simulink model "FOC_SMPMSM_SPWM"  (R2019a)
settings: Solver=VariableStepAuto  StartTime=0.0  StopTime=1  RelTol=1e-3
values from neighbouring files (symbols this model uses):
  Lq = 0.000165    [FOC_Parameters.mat]
  PM_flux = 0.11    [FOC_Parameters.mat]
  pp = 4    [FOC_Parameters.mat]
  Rs = 0.016    [FOC_Parameters.mat]
libraries: simulink x4, powerlib x3, electricdrivelib x1, powerlib_meascontrol x1
settings Model: Creator=ryusl  LastModifiedBy=ryusl

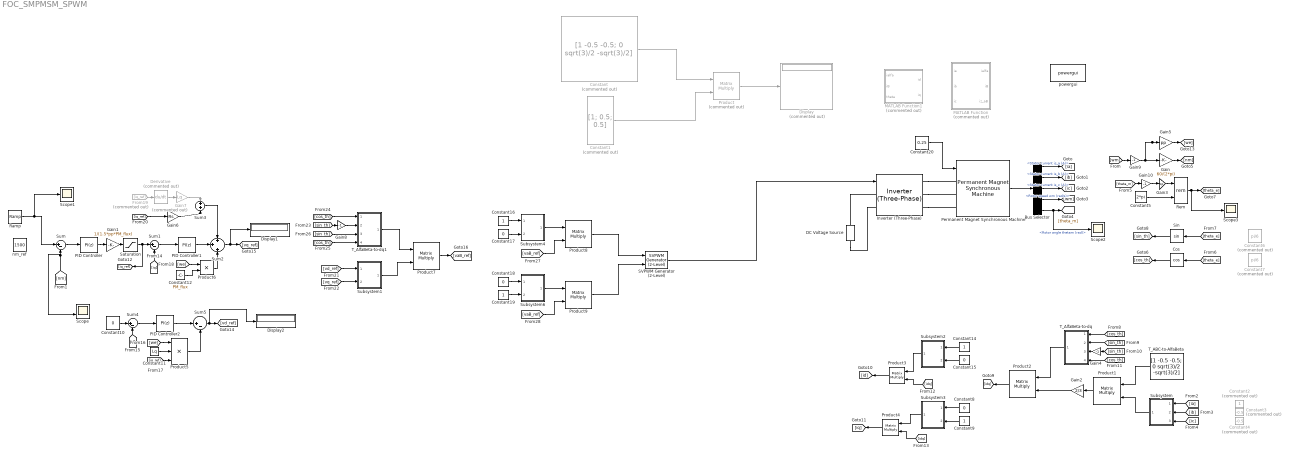
== system FOC_SMPMSM_SPWM ==
  Bus Selector : BusSelector  OutputSignals=Stator current is_a (A),Stator current is_b (A),Stator current is_c (A),Rotor speed wm (rad/s),Rotor angle thetam (rad)
  Constant : Constant  Commented=on  Value=[1 -0.5 -0.5; 0 sqrt(3)/2 -sqrt(3)/2]  VectorParams1D=off
  Constant1 : Constant  Commented=on  Value=[1; 0.5; 0.5]  VectorParams1D=off
  Constant{8,10,15,17..18} (5 alike) : Constant  Value=0
  Constant11 : Constant  Value=Lq
  Constant12 : Constant  Value=PM_flux
  Constant{9,14,16,19} (4 alike) : Constant
  Constant2 : Constant  Commented=on
  Constant20 : Constant  Value=0.25
  Constant3 : Constant  Commented=on  Value=-0.5
  Constant4 : Constant  Commented=on  Value=-0.5
  Constant5 : Constant  Value=2*pi
  Constant6 : Constant  Commented=on  Value=pi/6
  Constant7 : Constant  Commented=on  Value=pi/6
  Cos : Trigonometry  Operator=cos
  DC Voltage Source : powerlib/Electrical Sources/DC Voltage Source  Amplitude=600  Measurements=None
      settings: SourceProductName=Simscape Electrical
  Derivative : Derivative  Commented=on
  Display : Display  Commented=on
  Display1 : Display
  Display2 : Display
  From19 : From  Commented=on  GotoTag=iq_ref
  Gain : Gain  Gain=60/(2*pi)
  Gain1 : Gain  Gain=1/(1.5*pp*PM_flux)
  Gain{4,8..10} (4 alike) : Gain  Gain=-1
  Gain2 : Gain  Gain=2/3
  Gain3 : Gain  Gain=pp
  Gain5 : Gain  Gain=pp
  Gain6 : Gain  Gain=Rs
  Gain7 : Gain  Commented=on  Gain=Lq
  Inverter (Three-Phase) : electricdrivelib/Fundamental Drive Blocks/Inverter (Three-Phase)  LabelModeActiveChoice=Detailed  detailLevel=Detailed  driveType=Field-oriented control  Ts=2e-6  SnubberResistance=10e3  SnubberCapacitance=inf  Device=IGBT / Diodes  Ron=1e-3  ForwardVoltages=[1.2,1.2]  GTOparameters=[1e-6,2e-6]  IGBTparameters=[1e-6,2e-6]  Measurements=All voltages and currents  converterType=Inverter  SourceFrequency=60  ReferenceFrame=Rotor  dqInductances=[8.5e-3,8.5e-3]  Inductance=8.5e-3  Ls=0  Resistance=0.2  Flux=0.175  Stator_sm=[2.01e-3,4.289e-4,4.477e-3,1.354e-3]  Stator_im=[14.85e-3,0.3027e-3]  Rotor=[9.295e-3,0.3027e-3]  Lm=10.46e-3  p=4
      settings: AttributesFormatString=%<BlockChoice>  SourceProductName=Simscape Electrical  SourceProductBaseCode=PS
  MATLAB Function : MATLAB Function  Commented=on  TreatAsAtomicUnit=on
  MATLAB Function1 : MATLAB Function  Commented=on  TreatAsAtomicUnit=on
  PID Controller : simulink/Continuous/PID Controller  Controller=PI  Form=Parallel  TimeDomain=Discrete-time  SampleTime=-1  IntegratorMethod=Forward Euler  FilterMethod=Forward Euler  ControllerParametersSource=internal  P=10  I=2  D=0  UseFilter=on  N=100  TunerSelectOption=Transfer Function Based (PID Tuner App)  InitialConditionSource=internal  InitialConditionForIntegrator=0  InitialConditionForFilter=0  DifferentiatorICPrevScaledInput=0  ExternalReset=none  TrackingMode=off  Kt=1  LimitOutput=off  UpperSaturationLimit=inf  LowerSaturationLimit=-inf  LinearizeAsGain=on  AntiWindupMode=none  Kb=1  POutMin=[]  POutMax=[]  IOutMin=[]  IOutMax=[]  DOutMin=[]  DOutMax=[]  NOutMin=[]  NOutMax=[]  SumOutMin=[]  SumOutMax=[]  SaturationOutMin=[]  SaturationOutMax=[]  PParamMin=[]  PParamMax=[]  IParamMin=[]  IParamMax=[]  DParamMin=[]  DParamMax=[]  NParamMin=[]  NParamMax=[]  KbParamMin=[]  KbParamMax=[]  KtParamMin=[]  KtParamMax=[]  KbOutMin=[]  KbOutMax=[]  KtOutMin=[]  KtOutMax=[]  IntegratorOutMin=[]  IntegratorOutMax=[]  FilterOutMin=[]  FilterOutMax=[]  SumI1OutMin=[]  SumI1OutMax=[]  SumI2OutMin=[]  SumI2OutMax=[]  SumI3OutMin=[]  SumI3OutMax=[]  SumI4OutMin=[]  SumI4OutMax=[]  SumDOutMin=[]  SumDOutMax=[]  DifferentiatorOutMin=[]  DifferentiatorOutMax=[]  FilterDiffOutCoefMin=[]  FilterDiffOutCoefMax=[]  ReciprocalOutMin=[]  ReciprocalOutMax=[]  SumDenOutMin=[]  SumDenOutMax=[]  SumNumOutMin=[]  SumNumOutMax=[]  DivideOutMin=[]  DivideOutMax=[]  IntegratorContinuousStateAttributes=''  IntegratorStateMustResolveToSignalObject=off  IntegratorRTWStateStorageClass=Auto  FilterContinuousStateAttributes=''  FilterStateMustResolveToSignalObject=off  FilterRTWStateStorageClass=Auto  ParallelPVariant=InternalParameters  IdealPVariant=Disabled  IVariant=InternalParameters  DVariant=Disabled  IntegratorVariant=Discrete  SatVariant=Disabled  AWVariant=Passthrough  PCopyVariant=Disabled  TRVariant=Disabled  FdbkBlocksVariant=Forward  IdealPFdbkVariant=Disabled  SatFdbkVariant=Disabled  DerivativeFilterVariant=Disabled  NVariant=Disabled  NCopyVariant=Disabled_SignalSpec  FilterICVariant=Disabled  IntegratorICVariant=InternalICs  ExternalResetVariant=Disabled  TRSumVariant=Passthrough  SumFdbkVariant=Disabled  SumVariant=Sum_PI
  PID Controller1 : simulink/Continuous/PID Controller  Controller=PI  Form=Parallel  TimeDomain=Discrete-time  SampleTime=-1  IntegratorMethod=Forward Euler  FilterMethod=Forward Euler  ControllerParametersSource=internal  P=5  I=0.5  D=0  UseFilter=on  N=100  TunerSelectOption=Transfer Function Based (PID Tuner App)  InitialConditionSource=internal  InitialConditionForIntegrator=0  InitialConditionForFilter=0  DifferentiatorICPrevScaledInput=0  ExternalReset=none  TrackingMode=off  Kt=1  LimitOutput=off  UpperSaturationLimit=inf  LowerSaturationLimit=-inf  LinearizeAsGain=on  AntiWindupMode=none  Kb=1  POutMin=[]  POutMax=[]  IOutMin=[]  IOutMax=[]  DOutMin=[]  DOutMax=[]  NOutMin=[]  NOutMax=[]  SumOutMin=[]  SumOutMax=[]  SaturationOutMin=[]  SaturationOutMax=[]  PParamMin=[]  PParamMax=[]  IParamMin=[]  IParamMax=[]  DParamMin=[]  DParamMax=[]  NParamMin=[]  NParamMax=[]  KbParamMin=[]  KbParamMax=[]  KtParamMin=[]  KtParamMax=[]  KbOutMin=[]  KbOutMax=[]  KtOutMin=[]  KtOutMax=[]  IntegratorOutMin=[]  IntegratorOutMax=[]  FilterOutMin=[]  FilterOutMax=[]  SumI1OutMin=[]  SumI1OutMax=[]  SumI2OutMin=[]  SumI2OutMax=[]  SumI3OutMin=[]  SumI3OutMax=[]  SumI4OutMin=[]  SumI4OutMax=[]  SumDOutMin=[]  SumDOutMax=[]  DifferentiatorOutMin=[]  DifferentiatorOutMax=[]  FilterDiffOutCoefMin=[]  FilterDiffOutCoefMax=[]  ReciprocalOutMin=[]  ReciprocalOutMax=[]  SumDenOutMin=[]  SumDenOutMax=[]  SumNumOutMin=[]  SumNumOutMax=[]  DivideOutMin=[]  DivideOutMax=[]  IntegratorContinuousStateAttributes=''  IntegratorStateMustResolveToSignalObject=off  IntegratorRTWStateStorageClass=Auto  FilterContinuousStateAttributes=''  FilterStateMustResolveToSignalObject=off  FilterRTWStateStorageClass=Auto  ParallelPVariant=InternalParameters  IdealPVariant=Disabled  IVariant=InternalParameters  DVariant=Disabled  IntegratorVariant=Discrete  SatVariant=Disabled  AWVariant=Passthrough  PCopyVariant=Disabled  TRVariant=Disabled  FdbkBlocksVariant=Forward  IdealPFdbkVariant=Disabled  SatFdbkVariant=Disabled  DerivativeFilterVariant=Disabled  NVariant=Disabled  NCopyVariant=Disabled_SignalSpec  FilterICVariant=Disabled  IntegratorICVariant=InternalICs  ExternalResetVariant=Disabled  TRSumVariant=Passthrough  SumFdbkVariant=Disabled  SumVariant=Sum_PI
  PID Controller2 : simulink/Continuous/PID Controller  Controller=PI  Form=Parallel  TimeDomain=Discrete-time  SampleTime=-1  IntegratorMethod=Forward Euler  FilterMethod=Forward Euler  ControllerParametersSource=internal  P=5  I=0.5  D=0  UseFilter=on  N=100  TunerSelectOption=Transfer Function Based (PID Tuner App)  InitialConditionSource=internal  InitialConditionForIntegrator=0  InitialConditionForFilter=0  DifferentiatorICPrevScaledInput=0  ExternalReset=none  TrackingMode=off  Kt=1  LimitOutput=off  UpperSaturationLimit=inf  LowerSaturationLimit=-inf  LinearizeAsGain=on  AntiWindupMode=none  Kb=1  POutMin=[]  POutMax=[]  IOutMin=[]  IOutMax=[]  DOutMin=[]  DOutMax=[]  NOutMin=[]  NOutMax=[]  SumOutMin=[]  SumOutMax=[]  SaturationOutMin=[]  SaturationOutMax=[]  PParamMin=[]  PParamMax=[]  IParamMin=[]  IParamMax=[]  DParamMin=[]  DParamMax=[]  NParamMin=[]  NParamMax=[]  KbParamMin=[]  KbParamMax=[]  KtParamMin=[]  KtParamMax=[]  KbOutMin=[]  KbOutMax=[]  KtOutMin=[]  KtOutMax=[]  IntegratorOutMin=[]  IntegratorOutMax=[]  FilterOutMin=[]  FilterOutMax=[]  SumI1OutMin=[]  SumI1OutMax=[]  SumI2OutMin=[]  SumI2OutMax=[]  SumI3OutMin=[]  SumI3OutMax=[]  SumI4OutMin=[]  SumI4OutMax=[]  SumDOutMin=[]  SumDOutMax=[]  DifferentiatorOutMin=[]  DifferentiatorOutMax=[]  FilterDiffOutCoefMin=[]  FilterDiffOutCoefMax=[]  ReciprocalOutMin=[]  ReciprocalOutMax=[]  SumDenOutMin=[]  SumDenOutMax=[]  SumNumOutMin=[]  SumNumOutMax=[]  DivideOutMin=[]  DivideOutMax=[]  IntegratorContinuousStateAttributes=''  IntegratorStateMustResolveToSignalObject=off  IntegratorRTWStateStorageClass=Auto  FilterContinuousStateAttributes=''  FilterStateMustResolveToSignalObject=off  FilterRTWStateStorageClass=Auto  ParallelPVariant=InternalParameters  IdealPVariant=Disabled  IVariant=InternalParameters  DVariant=Disabled  IntegratorVariant=Discrete  SatVariant=Disabled  AWVariant=Passthrough  PCopyVariant=Disabled  TRVariant=Disabled  FdbkBlocksVariant=Forward  IdealPFdbkVariant=Disabled  SatFdbkVariant=Disabled  DerivativeFilterVariant=Disabled  NVariant=Disabled  NCopyVariant=Disabled_SignalSpec  FilterICVariant=Disabled  IntegratorICVariant=InternalICs  ExternalResetVariant=Disabled  TRSumVariant=Passthrough  SumFdbkVariant=Disabled  SumVariant=Sum_PI
  Permanent Magnet Synchronous Machine : powerlib/Machines/Permanent Magnet Synchronous Machine  NbPhases=3  FluxDistribution=Sinusoidal  RotorType=Round  MechanicalLoad=Torque Tm  PresetModel=No  ShowDetailedParameters=on  MeasurementBus=off  Resistance=Rs  Inductance=8.5e-3  dqInductances=[8.5e-3,8.5e-3]  La=Ld  MachineConstant=Flux linkage established by magnets (V.s)  Flux=PM_flux  VoltageCst=79.8072  TorqueCst=0.66  Flat=120  Mechanical=[0.0027 0.0004924 pp 0]  PolePairs=4  InitialConditions=[0,0, 0,0]  InitialConditions5ph=[0 0 0 0 0 0]  TsPowergui=0  TsBlock=-1  RefAngle=90 degrees behind phase A axis (modified Park)
  Product : Product  Commented=on  Multiplication=Matrix(*)
  Product{1..4,7..9} (7 alike) : Product  Multiplication=Matrix(*)
  Product5 : Product  Inputs=3
  Product6 : Product
  Ramp : simulink/Sources/Ramp  slope=1000  start=0  InitialOutput=0
  Rem : Math  Operator=rem  SaturateOnIntegerOverflow=on
  SVPWM Generator (2-Level) : powerlib_meascontrol/Pulse & Signal Generators/SVPWM Generator (2-Level)  InputType=alpha-beta components  SwitchingPattern=Pattern #1  Fc=2000  ParUref=[0.8 -30 50]  Ts=0
      settings: SourceProductName=Simscape Electrical  SourceProductBaseCode=PS
  Saturation : Saturate  UpperLimit=500  LowerLimit=0
  Scope : Scope  NumInputPorts=2
  Scope1 : Scope
  Scope2 : Scope
  Scope3 : Scope
  Sin : Trigonometry
  Subsystem : Subsystem
  Subsystem1 : Subsystem
  Subsystem2 : Subsystem
  Subsystem3 : Subsystem
  Subsystem4 : Subsystem
  Subsystem6 : Subsystem
  Sum{,1,4..5} (4 alike) : Sum  Inputs=|+-
  Sum2 : Sum  Inputs=+|+|+
  Sum3 : Sum  Inputs=+|+
  T_ABC-to-AlfaBeta : Constant  Value=[1 -0.5 -0.5; 0 sqrt(3)/2 -sqrt(3)/2]  VectorParams1D=off
  T_AlfaBeta-to-dq : Subsystem
  T_AlfaBeta-to-dq1 : Subsystem
  nm_ref : Constant  Value=1500
  powergui : powerlib/powergui  Priority=1  SimulationMode=Discrete  SampleTime=1e-6  frequency=60  Iterations=50  frequencyindice=0  Pbase=100e6  ErrMax=1e-4  UnitsV=kV  UnitsW=MW  buscounter=0  FunctionMessages=off  echomessages=off  EnableUseOfTLC=off  CurrentSourceSwitches=off  DisableSnubberDevices=off  DisableRonSwitches=off  DisableVfSwitches=off  DisplayEquations=off  AutomaticDiscreteSolvers=off  SolverType=Tustin/Backward Euler (TBE)  Interpol=off  ExternalGateDelay=off  methode=off  Ts=100  x0status=blocks  SPID=on  SwTol=0  HookPort=off  NonlinearTolerance=0  nMaxIteration=15  ContinueOnMaxIteration=off  RestoreLinks=warning  ResistiveCurrentMeasurement=off  Frange=[0:2:500]  Ylog=off  Xlog=on  ShowGrid=off  save=off  variable=ZData  structure=0  ZoomFFT=off  StartTime=0.0  cycles=1  DisplayStyle=1  fundamental=60  FreqAxis=off  MaxFrequency=1000  frequencyindicesteady=1  RmsSteady=1  display=off
      settings: SourceProductName=Simscape Electrical
  wires:
  Constant/1 -> Product/1
  Constant1/1 -> Product/2
  Product/1 -> Display/1
  Permanent Magnet Synchronous Machine/1 -> Bus Selector/1
  Bus Selector/1 -> [ia]  "<Stator current is_a (A)>"
  Bus Selector/2 -> [ib]  "<Stator current is_b (A)>"
  Bus Selector/3 -> [ic]  "<Stator current is_c (A)>"
  Bus Selector/4 -> [wm]  "<Rotor speed wm (rad/s)>"
  Bus Selector/5 -> Scope2/1, [theta_m]  "<Rotor angle thetam (rad)>"
  Gain/1 -> [nm]
  Sum/1 -> PID Controller/1
  [nm] -> Scope/2, Sum/2
  PID Controller/1 -> Gain1/1
  T_ABC-to-AlfaBeta/1 -> Product1/1
  Subsystem/1(Matrix) -> Product1/2
  Product1/1 -> Gain2/1
  Constant5/1 -> Rem/2
  Gain3/1 -> Rem/1
  Rem/1 -> Scope3/1, [theta_e]
  Cos/1 -> [cos_th]
  Sin/1 -> [sin_th]
  Gain4/1 -> T_AlfaBeta-to-dq/3(M21)
  [cos_th] -> T_AlfaBeta-to-dq/1(M11)
  [sin_th] -> T_AlfaBeta-to-dq/2(M12)
  [sin_th] -> Gain4/1
  [cos_th] -> T_AlfaBeta-to-dq/4("M22 ")
  Gain2/1 -> Product2/2
  T_AlfaBeta-to-dq/1(Matrix) -> Product2/1
  Product2/1 -> [idq]
  [idq] -> Product3/2
  Product3/1 -> [id]
  Product4/1 -> [iq]
  [iq] -> Sum1/2
  Sum1/1 -> PID Controller1/1
  PID Controller1/1 -> Sum2/2
  Gain5/1 -> [we]
  Sum4/1 -> PID Controller2/1
  [id] -> Sum4/2
  Constant10/1 -> Sum4/1
  [iq_ref] -> Product5/3
  Constant11/1 -> Product5/2
  [we] -> Product5/1
  Product5/1 -> Sum5/2
  PID Controller2/1 -> Sum5/1
  Sum5/1 -> Display2/1, [vd_ref]
  Product6/1 -> Sum2/3
  [we] -> Product6/1
  Constant12/1 -> Product6/2
  From19/1 -> Derivative/1
  [iq_ref] -> Gain6/1
  Gain6/1 -> Sum3/2
  Derivative/1 -> Gain7/1
  Gain7/1 -> Sum3/1
  Sum3/1 -> Sum2/1
  Sum2/1 -> Display1/1, [vq_ref]
  [vq_ref] -> Subsystem1/2(M21)
  [vd_ref] -> Subsystem1/1(M11)
  Constant14/1 -> Subsystem2/1(M11)
  Constant15/1 -> Subsystem2/2(M21)
  Subsystem2/1(Matrix) -> Product3/1
  Constant8/1 -> Subsystem3/1(M11)
  Constant9/1 -> Subsystem3/2(M21)
  Subsystem3/1(Matrix) -> Product4/1
  [idq] -> Product4/2
  [sin_th] -> Gain8/1
  Gain8/1 -> T_AlfaBeta-to-dq1/2(M12)
  [cos_th] -> T_AlfaBeta-to-dq1/1(M11)
  [sin_th] -> T_AlfaBeta-to-dq1/3(M21)
  [cos_th] -> T_AlfaBeta-to-dq1/4("M22 ")
  T_AlfaBeta-to-dq1/1(Matrix) -> Product7/1
  Subsystem1/1(Matrix) -> Product7/2
  Constant17/1 -> Subsystem4/2(M21)
  Constant16/1 -> Subsystem4/1(M11)
  Subsystem4/1(Matrix) -> Product8/1
  [vaB_ref] -> Product8/2
  [vaB_ref] -> Product9/2
  Subsystem6/1(Matrix) -> Product9/1
  Constant18/1 -> Subsystem6/1(M11)
  Constant19/1 -> Subsystem6/2(M21)
  Product7/1 -> [vaB_ref]
  Product8/1 -> SVPWM Generator (2-Level)/1
  Product9/1 -> SVPWM Generator (2-Level)/2
  Constant20/1 -> Permanent Magnet Synchronous Machine/1
  [theta_e] -> Sin/1
  [theta_e] -> Cos/1
  [ia] -> Subsystem/1(M11)
  [ib] -> Subsystem/2(M21)
  [ic] -> Subsystem/3(M31)
  Gain1/1 -> Saturation/1
  Saturation/1 -> [iq_ref], Sum1/1
  Ramp/1 -> Scope1/1, Sum/1
  SVPWM Generator (2-Level)/1 -> Inverter (Three-Phase)/1
  [wm] -> Gain9/1
  Gain9/1 -> Gain5/1, Gain/1
  [theta_m] -> Gain10/1
  Gain10/1 -> Gain3/1
  connections:
  Inverter (Three-Phase)/RConn1 -- Permanent Magnet Synchronous Machine/LConn1
  Inverter (Three-Phase)/RConn2 -- Permanent Magnet Synchronous Machine/LConn2
  Inverter (Three-Phase)/RConn3 -- Permanent Magnet Synchronous Machine/LConn3
  DC Voltage Source/RConn1 -- Inverter (Three-Phase)/LConn1
  DC Voltage Source/LConn1 -- Inverter (Three-Phase)/LConn2

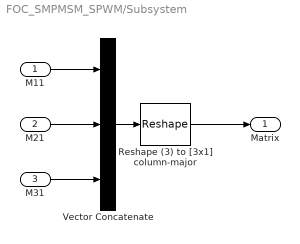
== system FOC_SMPMSM_SPWM/Subsystem ==
  M11 : Inport  PortDimensions=1
  M21 : Inport  Port=2  PortDimensions=1
  M31 : Inport  Port=3  PortDimensions=1
  Reshape (3) to [3x1] column-major : Reshape  OutputDimensionality=Customize  OutputDimensions=[3,1]
  Vector Concatenate : Concatenate  NumInputs=3
  Matrix : Outport  PortDimensions=[3 1]
  wires:
  M11/1 -> Vector Concatenate/1
  Vector Concatenate/1 -> Reshape (3) to [3x1] column-major/1
  M21/1 -> Vector Concatenate/2
  Reshape (3) to [3x1] column-major/1 -> Matrix/1
  M31/1 -> Vector Concatenate/3

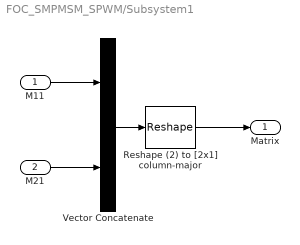
== system FOC_SMPMSM_SPWM/Subsystem1 ==
  M11 : Inport  PortDimensions=1
  M21 : Inport  Port=2  PortDimensions=1
  Reshape (2) to [2x1] column-major : Reshape  OutputDimensionality=Customize  OutputDimensions=[2,1]
  Vector Concatenate : Concatenate
  Matrix : Outport  PortDimensions=[2 1]
  wires:
  Reshape (2) to [2x1] column-major/1 -> Matrix/1
  M21/1 -> Vector Concatenate/2
  Vector Concatenate/1 -> Reshape (2) to [2x1] column-major/1
  M11/1 -> Vector Concatenate/1

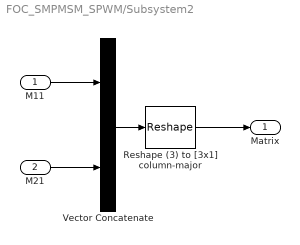
== system FOC_SMPMSM_SPWM/Subsystem2 ==
  M11 : Inport  PortDimensions=1
  M21 : Inport  Port=2  PortDimensions=1
  Reshape (3) to [3x1] column-major : Reshape  OutputDimensionality=Customize  OutputDimensions=[1,2]
  Vector Concatenate : Concatenate
  Matrix : Outport  PortDimensions=[1 2]
  wires:
  M11/1 -> Vector Concatenate/1
  Vector Concatenate/1 -> Reshape (3) to [3x1] column-major/1
  M21/1 -> Vector Concatenate/2
  Reshape (3) to [3x1] column-major/1 -> Matrix/1

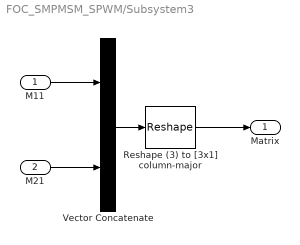
== system FOC_SMPMSM_SPWM/Subsystem3 ==
  M11 : Inport  PortDimensions=1
  M21 : Inport  Port=2  PortDimensions=1
  Reshape (3) to [3x1] column-major : Reshape  OutputDimensionality=Customize  OutputDimensions=[1,2]
  Vector Concatenate : Concatenate
  Matrix : Outport  PortDimensions=[1 2]
  wires:
  M11/1 -> Vector Concatenate/1
  Vector Concatenate/1 -> Reshape (3) to [3x1] column-major/1
  M21/1 -> Vector Concatenate/2
  Reshape (3) to [3x1] column-major/1 -> Matrix/1

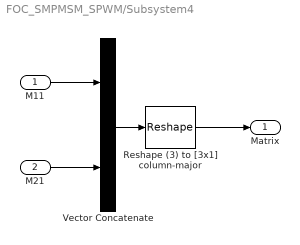
== system FOC_SMPMSM_SPWM/Subsystem4 ==
  M11 : Inport  PortDimensions=1
  M21 : Inport  Port=2  PortDimensions=1
  Reshape (3) to [3x1] column-major : Reshape  OutputDimensionality=Customize  OutputDimensions=[1,2]
  Vector Concatenate : Concatenate
  Matrix : Outport  PortDimensions=[1 2]
  wires:
  Reshape (3) to [3x1] column-major/1 -> Matrix/1
  M21/1 -> Vector Concatenate/2
  Vector Concatenate/1 -> Reshape (3) to [3x1] column-major/1
  M11/1 -> Vector Concatenate/1

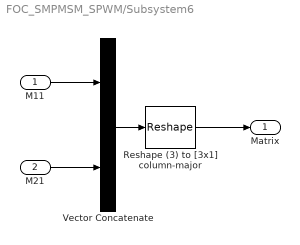
== system FOC_SMPMSM_SPWM/Subsystem6 ==
  M11 : Inport  PortDimensions=1
  M21 : Inport  Port=2  PortDimensions=1
  Reshape (3) to [3x1] column-major : Reshape  OutputDimensionality=Customize  OutputDimensions=[1,2]
  Vector Concatenate : Concatenate
  Matrix : Outport  PortDimensions=[1 2]
  wires:
  M11/1 -> Vector Concatenate/1
  Vector Concatenate/1 -> Reshape (3) to [3x1] column-major/1
  M21/1 -> Vector Concatenate/2
  Reshape (3) to [3x1] column-major/1 -> Matrix/1

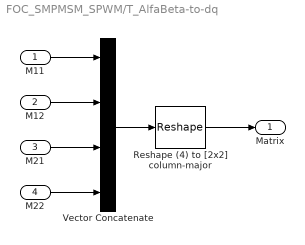
== system FOC_SMPMSM_SPWM/T_AlfaBeta-to-dq ==
  M11 : Inport  PortDimensions=1
  M12 : Inport  Port=2  PortDimensions=1
  M21 : Inport  Port=3  PortDimensions=1
  "M22 " : Inport  Port=4  PortDimensions=1
  Reshape (4) to [2x2] column-major : Reshape  OutputDimensionality=Customize  OutputDimensions=[2,2]
  Vector Concatenate : Concatenate  NumInputs=4
  Matrix : Outport  PortDimensions=[2 2]
  wires:
  M21/1 -> Vector Concatenate/3
  Reshape (4) to [2x2] column-major/1 -> Matrix/1
  M12/1 -> Vector Concatenate/2
  Vector Concatenate/1 -> Reshape (4) to [2x2] column-major/1
  M11/1 -> Vector Concatenate/1
  "M22 "/1 -> Vector Concatenate/4

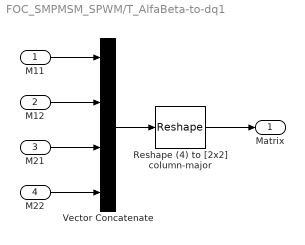
== system FOC_SMPMSM_SPWM/T_AlfaBeta-to-dq1 ==
  M11 : Inport  PortDimensions=1
  M12 : Inport  Port=2  PortDimensions=1
  M21 : Inport  Port=3  PortDimensions=1
  "M22 " : Inport  Port=4  PortDimensions=1
  Reshape (4) to [2x2] column-major : Reshape  OutputDimensionality=Customize  OutputDimensions=[2,2]
  Vector Concatenate : Concatenate  NumInputs=4
  Matrix : Outport  PortDimensions=[2 2]
  wires:
  M21/1 -> Vector Concatenate/3
  Reshape (4) to [2x2] column-major/1 -> Matrix/1
  M12/1 -> Vector Concatenate/2
  Vector Concatenate/1 -> Reshape (4) to [2x2] column-major/1
  M11/1 -> Vector Concatenate/1
  "M22 "/1 -> Vector Concatenate/4

== matlab function FOC_SMPMSM_SPWM/MATLAB Function1 ==
  data: ialfa input; id output; iB input; theta input; iq output
function [id,iq] = aB_dq(ialfa,iB,theta)
T_aB-dq = [cos(theta) sin(theta); -sin(theta) cos(theta)];
[id,iq] = T_ab-dq*[ialfa; iB];

== matlab function FOC_SMPMSM_SPWM/MATLAB Function ==
  data: ialfa output; ia input; ib input; ic input; iB output; iz_aB output
function [ialfa,iB,iz_aB] = abc_aB(ia,ib,ic)
T_abc_aB = (2/3).*[1 -0.5 -0.5; 0 sqrt(3)/2 -sqrt(3)/2; 0.5 0.5 0.5];
[ialfa,iB,iz_aB] = T_abc_aB*[ia; ib; ic];
